simulink model "EKF_SIL_02_newdelIps"  (R2015a)
settings: Solver=ode45  StartTime=0.0  StopTime=totalSimulationTime  RelTol=1e-3
model workspace: external: MATLAB File Init_Model_02_Simulink_SIL1.m (data not in the file)
values from neighbouring files (symbols this model uses):
  Cov_nu = [0.005 0 0 0 ... (first row only)    [InitOOSM.m]    (also in InitSIL.m; Init_Model_02_Simulink.m; Init_Model_02_Simulink_SIL1.m)
  Cov_r = [0.003 0 0 ... (first row only)    [InitOOSM.m]    (also in InitSIL.m; Init_Model_02_Simulink.m; Init_Model_02_Simulink_SIL1.m)
  e_force_x = 0    [InitOOSM.m]    (also in InitSIL.m; Init_Model_02_Simulink.m; Init_Model_02_Simulink_SIL1.m)
  e_force_y = 0    [InitOOSM.m]    (also in InitSIL.m; Init_Model_02_Simulink.m; Init_Model_02_Simulink_SIL1.m)
  e_force_z = 0    [InitOOSM.m]    (also in InitSIL.m; Init_Model_02_Simulink.m; Init_Model_02_Simulink_SIL1.m)
  ieps = [-0.7071;0;0;0.7071]    [InitOOSM.m]    (also in InitSIL.m; Init_Model_02_Simulink.m = [-0.7071; 0; 0; 0.7071]; Init_Model_02_Simulink_SIL1.m)
  ita = [0.5;0.5;0.5;0.5]    [InitOOSM.m]    (also in InitSIL.m; Init_Model_02_Simulink.m = [0.5; 0.5; 0.5; 0.5]; Init_Model_02_Simulink_SIL1.m)
  n = 0.00    (= 0)    [InitOOSM.m]    (also in InitSIL.m; Init_Model_02_Simulink.m; Init_Model_02_Simulink_SIL1.m)
  P_0 = 0.5*eye(18,18)    [InitOOSM.m]    (also in InitSIL.m = 0.05*eye(12,12); Init_Model_02_Simulink.m = 0.005*eye(12,12); Init_Model_02_Simulink_SIL1.m = 0.005*eye(12,12))
  p_x = 0.75    [InitOOSM.m]    (also in InitSIL.m; Init_Model_02_Simulink.m; Init_Model_02_Simulink_SIL1.m)
  p_y = 0.125    [InitOOSM.m]    (also in InitSIL.m; Init_Model_02_Simulink.m; Init_Model_02_Simulink_SIL1.m)
  p_z = -0.8    [InitOOSM.m]    (also in InitSIL.m; Init_Model_02_Simulink.m; Init_Model_02_Simulink_SIL1.m)
  parameter_gravitation = 3.986005E+14    (= 398600500000000)    [InitOOSM.m]    (also in InitSIL.m; Init_Model_02_Simulink.m; Init_Model_02_Simulink_SIL1.m)
  rho = [0.04;0;0.3]    [InitOOSM.m]    (also in InitSIL.m; Init_Model_02_Simulink.m = [0.04; 0; 0.3]; Init_Model_02_Simulink_SIL1.m)
  rho_c = [-0.00017;   -0.9780;   -0.1854]    [InitOOSM.m]    (also in InitSIL.m = [0.00036;   -0.9865;   -0.1854]; Init_Model_02_Simulink.m = [0.00036; -0.9865; -0.1854]; Init_Model_02_Simulink_SIL1.m = [0.00036;   -0.9865;   -0.1854])
  sig_f = 2E-6    (= 2e-06)    [InitOOSM.m]    (also in InitSIL.m; Init_Model_02_Simulink.m; Init_Model_02_Simulink_SIL1.m)
  sig_tau = 2.5E-5    (= 2.5e-05)    [InitOOSM.m]    (also in InitSIL.m; Init_Model_02_Simulink.m; Init_Model_02_Simulink_SIL1.m)
  t_delta = 0.2    [InitOOSM.m]    (also in InitSIL.m; Init_Model_02_Simulink.m; Init_Model_02_Simulink_SIL1.m)
  t_Kalman = 0.01    [InitOOSM.m]    (also in InitSIL.m; Init_Model_02_Simulink.m; Init_Model_02_Simulink_SIL1.m)
  t_RobotSense = 0.05    [InitOOSM.m]    (also in InitSIL.m; Init_Model_02_Simulink.m; Init_Model_02_Simulink_SIL1.m)
  tau_1 = 0    [InitOOSM.m]    (also in InitSIL.m; Init_Model_02_Simulink.m; Init_Model_02_Simulink_SIL1.m)
  tau_2 = 0    [InitOOSM.m]    (also in InitSIL.m; Init_Model_02_Simulink.m; Init_Model_02_Simulink_SIL1.m)
  tau_3 = 0    [InitOOSM.m]    (also in InitSIL.m; Init_Model_02_Simulink.m; Init_Model_02_Simulink_SIL1.m)
  U_n_d = Simulink.Signal    [InitOOSM.m]    (also in InitSIL.m; Init_Model_02_Simulink.m; Init_Model_02_Simulink_SIL1.m)
  X_a_0 = [0; 0; 0; 1; 0; 0; 0; 0; 0; 0; 0; 0; 0;0;0;0;0;0;0;1]    [InitOOSM.m]    (also in InitSIL.m = [0; 0; 0; 1; 0; 0; 0; 0; 0; 0; 0; 0; 0]; Init_Model_02_Simulink.m = [0;0;0;0.707000000000000;0.707000000000000;0.200000000000000; Init_Model_02_Simulink_SIL1.m = [0;0;0.707;0.707;0.2;-0.02;0.0001;0.02;-1.80;0.50;-0.05;0.00)
libraries: simulink x5, dspmtrx3 x2, aerolibtransform2 x2, visionsinks x1
(part 4 of 4)

== system EKF_SIL_02_newdelIps/EKF/Predictor/Dynamic Model (Differential equations)2/Dynamic Model (Differential equations)/Orbital Dynamics /norm  ==
  vector : Inport
  Dot Product : DotProduct  InputSameDT=on  OutDataTypeStr=Inherit: Inherit via internal rule
  Sqrt : Sqrt  SaturateOnIntegerOverflow=on
  "norm " : Outport
  wires:
  Sqrt/1 -> "norm "/1
  vector/1 -> Dot Product/1, Dot Product/2
  Dot Product/1 -> Sqrt/1

== system EKF_SIL_02_newdelIps/EKF/Predictor/Dynamic Model (Differential equations)2/Dynamic Model (Differential equations)/Pose Servicer base//EE/Create Skew Symmetric ==
  vector : Inport
  0 : Constant  Value=0
  Create 3x3 matrix : Subsystem
  Demux : Demux  Outputs=3
  Demux1 : Demux  Outputs=3
  Gain : Gain  Gain=-1
  skew symmetric Matrix : Outport
  wires:
  0/1 -> Create 3x3 matrix/1(a11), Create 3x3 matrix/9(a33), Create 3x3 matrix/5(a22)
  Demux/3 -> Create 3x3 matrix/2(a12)
  Demux1/2 -> Create 3x3 matrix/3(a13)
  Demux1/3 -> Create 3x3 matrix/4(a21)
  Demux/1 -> Create 3x3 matrix/6(a23)
  vector/1 -> Demux1/1, Gain/1
  Create 3x3 matrix/1(Matrix) -> skew symmetric Matrix/1
  Gain/1 -> Demux/1
  Demux/2 -> Create 3x3 matrix/7(a31)
  Demux1/1 -> Create 3x3 matrix/8(a32)

== system EKF_SIL_02_newdelIps/EKF/Predictor/Dynamic Model (Differential equations)2/Dynamic Model (Differential equations)/Rotational Dynamics/Create  J ==
  p : Inport
  0 : Constant  Value=0  SampleTime=-1
  1 : Constant  SampleTime=-1
  Create 3x3 matrix : Subsystem
  Fcn : Fcn  Expr=1-u(2)/1+u(1)
  Fcn1 : Fcn  Expr=1+u(3)/1-u(1)
  "J_k " : Outport
  wires:
  1/1 -> Create 3x3 matrix/1(a11)
  Fcn1/1 -> Create 3x3 matrix/9(a33)
  Create 3x3 matrix/1(Matrix) -> "J_k "/1
  0/1 -> Create 3x3 matrix/2(a12), Create 3x3 matrix/3(a13), Create 3x3 matrix/4(a21), Create 3x3 matrix/6(a23), Create 3x3 matrix/7(a31), Create 3x3 matrix/8(a32)
  p/1 -> Fcn/1, Fcn1/1
  Fcn/1 -> Create 3x3 matrix/5(a22)

== system EKF_SIL_02_newdelIps/EKF/Predictor/Dynamic Model (Differential equations)2/Dynamic Model (Differential equations)/Rotational Dynamics/Create Psi ==
  "omega " : Inport
  p : Inport  Port=2
  Create Psi : Concatenate  NumInputs=3
  Demux : Demux  Outputs=3
  Demux1 : Demux  Outputs=3
  Product{,1..5} (6 alike) : Product
  Scope : Scope
      settings: SaveName=ScopeData20
  Psi : Outport
  wires:
  "omega "/1 -> Demux1/1
  Product3/1 -> Product2/2
  Product5/1 -> Product4/2
  Product1/1 -> Product/2
  Product/1 -> Create Psi/1
  Demux/2 -> Product2/1
  Create Psi/1 -> Psi/1, Scope/1
  Demux/1 -> Product/1
  Product2/1 -> Create Psi/2
  Demux1/2 -> Product5/1, Product1/1
  Demux1/1 -> Product3/1, Product5/2
  Product4/1 -> Create Psi/3
  Demux/3 -> Product4/1
  p/1 -> Demux/1
  Demux1/3 -> Product3/2, Product1/2

== system EKF_SIL_02_newdelIps/Plots and display/Create Measurements [Pose]1/Create Measurements [Position]/Create Rotation Matrix /Create Skew Symmetric/Create 3x3 matrix ==
  a11 : Inport
  a12 : Inport  Port=2
  a13 : Inport  Port=3
  a21 : Inport  Port=4
  a22 : Inport  Port=5
  a23 : Inport  Port=6
  a31 : Inport  Port=7
  a32 : Inport  Port=8
  a33 : Inport  Port=9
  Math Function : Math  Operator=transpose  SaturateOnIntegerOverflow=on
  Reshape (9) to [3x3] column-major : Reshape  OutputDimensionality=Customize  OutputDimensions=[3,3]
  Vector Concatenate : Concatenate  NumInputs=9
  Matrix : Outport
  wires:
  a33/1 -> Vector Concatenate/9
  a22/1 -> Vector Concatenate/5
  Vector Concatenate/1 -> Reshape (9) to [3x3] column-major/1
  a11/1 -> Vector Concatenate/1
  a12/1 -> Vector Concatenate/2
  a13/1 -> Vector Concatenate/3
  a23/1 -> Vector Concatenate/6
  a31/1 -> Vector Concatenate/7
  a32/1 -> Vector Concatenate/8
  a21/1 -> Vector Concatenate/4
  Reshape (9) to [3x3] column-major/1 -> Math Function/1
  Math Function/1 -> Matrix/1

== system EKF_SIL_02_newdelIps/Plots and display/Create Measurements [Pose]2/Create Measurements [Position]/Create Rotation Matrix /Create Skew Symmetric/Create 3x3 matrix ==
  a11 : Inport
  a12 : Inport  Port=2
  a13 : Inport  Port=3
  a21 : Inport  Port=4
  a22 : Inport  Port=5
  a23 : Inport  Port=6
  a31 : Inport  Port=7
  a32 : Inport  Port=8
  a33 : Inport  Port=9
  Math Function : Math  Operator=transpose  SaturateOnIntegerOverflow=on
  Reshape (9) to [3x3] column-major : Reshape  OutputDimensionality=Customize  OutputDimensions=[3,3]
  Vector Concatenate : Concatenate  NumInputs=9
  Matrix : Outport
  wires:
  Math Function/1 -> Matrix/1
  Reshape (9) to [3x3] column-major/1 -> Math Function/1
  a21/1 -> Vector Concatenate/4
  a32/1 -> Vector Concatenate/8
  a31/1 -> Vector Concatenate/7
  a23/1 -> Vector Concatenate/6
  a13/1 -> Vector Concatenate/3
  a12/1 -> Vector Concatenate/2
  a11/1 -> Vector Concatenate/1
  Vector Concatenate/1 -> Reshape (9) to [3x3] column-major/1
  a22/1 -> Vector Concatenate/5
  a33/1 -> Vector Concatenate/9

== system EKF_SIL_02_newdelIps/Plots and display/Create Measurements [Pose]2/Create Measurements [Position]/Create Rotation Matrix 1/Create Skew Symmetric/Create 3x3 matrix ==
  a11 : Inport
  a12 : Inport  Port=2
  a13 : Inport  Port=3
  a21 : Inport  Port=4
  a22 : Inport  Port=5
  a23 : Inport  Port=6
  a31 : Inport  Port=7
  a32 : Inport  Port=8
  a33 : Inport  Port=9
  Math Function : Math  Operator=transpose  SaturateOnIntegerOverflow=on
  Reshape (9) to [3x3] column-major : Reshape  OutputDimensionality=Customize  OutputDimensions=[3,3]
  Vector Concatenate : Concatenate  NumInputs=9
  Matrix : Outport
  wires:
  Math Function/1 -> Matrix/1
  Reshape (9) to [3x3] column-major/1 -> Math Function/1
  a21/1 -> Vector Concatenate/4
  a32/1 -> Vector Concatenate/8
  a31/1 -> Vector Concatenate/7
  a23/1 -> Vector Concatenate/6
  a13/1 -> Vector Concatenate/3
  a12/1 -> Vector Concatenate/2
  a11/1 -> Vector Concatenate/1
  Vector Concatenate/1 -> Reshape (9) to [3x3] column-major/1
  a22/1 -> Vector Concatenate/5
  a33/1 -> Vector Concatenate/9

== system EKF_SIL_02_newdelIps/EKF/Measurement Update/Update with K(k) and predict current state/Create H_k/Create Rotation Matrix /Create Skew Symmetric/Create 3x3 matrix ==
  a11 : Inport
  a12 : Inport  Port=2
  a13 : Inport  Port=3
  a21 : Inport  Port=4
  a22 : Inport  Port=5
  a23 : Inport  Port=6
  a31 : Inport  Port=7
  a32 : Inport  Port=8
  a33 : Inport  Port=9
  Math Function : Math  Operator=transpose  SaturateOnIntegerOverflow=on
  Reshape (9) to [3x3] column-major : Reshape  OutputDimensionality=Customize  OutputDimensions=[3,3]
  Vector Concatenate : Concatenate  NumInputs=9
  Matrix : Outport
  wires:
  a33/1 -> Vector Concatenate/9
  a22/1 -> Vector Concatenate/5
  Vector Concatenate/1 -> Reshape (9) to [3x3] column-major/1
  a11/1 -> Vector Concatenate/1
  a12/1 -> Vector Concatenate/2
  a13/1 -> Vector Concatenate/3
  a23/1 -> Vector Concatenate/6
  a31/1 -> Vector Concatenate/7
  a32/1 -> Vector Concatenate/8
  a21/1 -> Vector Concatenate/4
  Reshape (9) to [3x3] column-major/1 -> Math Function/1
  Math Function/1 -> Matrix/1

== system EKF_SIL_02_newdelIps/EKF/Measurement Update/Update with K(k) and predict current state/Create H_k/Create Rotation Matrix 1/Create Skew Symmetric/Create 3x3 matrix ==
  a11 : Inport
  a12 : Inport  Port=2
  a13 : Inport  Port=3
  a21 : Inport  Port=4
  a22 : Inport  Port=5
  a23 : Inport  Port=6
  a31 : Inport  Port=7
  a32 : Inport  Port=8
  a33 : Inport  Port=9
  Math Function : Math  Operator=transpose  SaturateOnIntegerOverflow=on
  Reshape (9) to [3x3] column-major : Reshape  OutputDimensionality=Customize  OutputDimensions=[3,3]
  Vector Concatenate : Concatenate  NumInputs=9
  Matrix : Outport
  wires:
  Math Function/1 -> Matrix/1
  Reshape (9) to [3x3] column-major/1 -> Math Function/1
  a21/1 -> Vector Concatenate/4
  a32/1 -> Vector Concatenate/8
  a31/1 -> Vector Concatenate/7
  a23/1 -> Vector Concatenate/6
  a13/1 -> Vector Concatenate/3
  a12/1 -> Vector Concatenate/2
  a11/1 -> Vector Concatenate/1
  Vector Concatenate/1 -> Reshape (9) to [3x3] column-major/1
  a22/1 -> Vector Concatenate/5
  a33/1 -> Vector Concatenate/9

== system EKF_SIL_02_newdelIps/EKF/Measurement Update/Update with K(k) and predict current state/Create H_k/Create Rotation Matrix 2/Create Skew Symmetric/Create 3x3 matrix ==
  a11 : Inport
  a12 : Inport  Port=2
  a13 : Inport  Port=3
  a21 : Inport  Port=4
  a22 : Inport  Port=5
  a23 : Inport  Port=6
  a31 : Inport  Port=7
  a32 : Inport  Port=8
  a33 : Inport  Port=9
  Math Function : Math  Operator=transpose  SaturateOnIntegerOverflow=on
  Reshape (9) to [3x3] column-major : Reshape  OutputDimensionality=Customize  OutputDimensions=[3,3]
  Vector Concatenate : Concatenate  NumInputs=9
  Matrix : Outport
  wires:
  a33/1 -> Vector Concatenate/9
  a22/1 -> Vector Concatenate/5
  Vector Concatenate/1 -> Reshape (9) to [3x3] column-major/1
  a11/1 -> Vector Concatenate/1
  a12/1 -> Vector Concatenate/2
  a13/1 -> Vector Concatenate/3
  a23/1 -> Vector Concatenate/6
  a31/1 -> Vector Concatenate/7
  a32/1 -> Vector Concatenate/8
  a21/1 -> Vector Concatenate/4
  Reshape (9) to [3x3] column-major/1 -> Math Function/1
  Math Function/1 -> Matrix/1

== system EKF_SIL_02_newdelIps/EKF/Measurement Update/Update with K(k) and predict current state/Create h/Create Rotation Matrix /Create Skew Symmetric/Create 3x3 matrix ==
  a11 : Inport
  a12 : Inport  Port=2
  a13 : Inport  Port=3
  a21 : Inport  Port=4
  a22 : Inport  Port=5
  a23 : Inport  Port=6
  a31 : Inport  Port=7
  a32 : Inport  Port=8
  a33 : Inport  Port=9
  Math Function : Math  Operator=transpose  SaturateOnIntegerOverflow=on
  Reshape (9) to [3x3] column-major : Reshape  OutputDimensionality=Customize  OutputDimensions=[3,3]
  Vector Concatenate : Concatenate  NumInputs=9
  Matrix : Outport
  wires:
  a33/1 -> Vector Concatenate/9
  a22/1 -> Vector Concatenate/5
  Vector Concatenate/1 -> Reshape (9) to [3x3] column-major/1
  a11/1 -> Vector Concatenate/1
  a12/1 -> Vector Concatenate/2
  a13/1 -> Vector Concatenate/3
  a23/1 -> Vector Concatenate/6
  a31/1 -> Vector Concatenate/7
  a32/1 -> Vector Concatenate/8
  a21/1 -> Vector Concatenate/4
  Reshape (9) to [3x3] column-major/1 -> Math Function/1
  Math Function/1 -> Matrix/1

== system EKF_SIL_02_newdelIps/EKF/Measurement Update/Update with K(k) and predict current state/Create h/Create Rotation Matrix 1/Create Skew Symmetric/Create 3x3 matrix ==
  a11 : Inport
  a12 : Inport  Port=2
  a13 : Inport  Port=3
  a21 : Inport  Port=4
  a22 : Inport  Port=5
  a23 : Inport  Port=6
  a31 : Inport  Port=7
  a32 : Inport  Port=8
  a33 : Inport  Port=9
  Math Function : Math  Operator=transpose  SaturateOnIntegerOverflow=on
  Reshape (9) to [3x3] column-major : Reshape  OutputDimensionality=Customize  OutputDimensions=[3,3]
  Vector Concatenate : Concatenate  NumInputs=9
  Matrix : Outport
  wires:
  a33/1 -> Vector Concatenate/9
  a22/1 -> Vector Concatenate/5
  Vector Concatenate/1 -> Reshape (9) to [3x3] column-major/1
  a11/1 -> Vector Concatenate/1
  a12/1 -> Vector Concatenate/2
  a13/1 -> Vector Concatenate/3
  a23/1 -> Vector Concatenate/6
  a31/1 -> Vector Concatenate/7
  a32/1 -> Vector Concatenate/8
  a21/1 -> Vector Concatenate/4
  Reshape (9) to [3x3] column-major/1 -> Math Function/1
  Math Function/1 -> Matrix/1

== system EKF_SIL_02_newdelIps/EKF/Measurement Update/Update with K(k) and predict current state/Create h/Create Rotation Matrix 2/Create Skew Symmetric/Create 3x3 matrix ==
  a11 : Inport
  a12 : Inport  Port=2
  a13 : Inport  Port=3
  a21 : Inport  Port=4
  a22 : Inport  Port=5
  a23 : Inport  Port=6
  a31 : Inport  Port=7
  a32 : Inport  Port=8
  a33 : Inport  Port=9
  Math Function : Math  Operator=transpose  SaturateOnIntegerOverflow=on
  Reshape (9) to [3x3] column-major : Reshape  OutputDimensionality=Customize  OutputDimensions=[3,3]
  Vector Concatenate : Concatenate  NumInputs=9
  Matrix : Outport
  wires:
  Math Function/1 -> Matrix/1
  Reshape (9) to [3x3] column-major/1 -> Math Function/1
  a21/1 -> Vector Concatenate/4
  a32/1 -> Vector Concatenate/8
  a31/1 -> Vector Concatenate/7
  a23/1 -> Vector Concatenate/6
  a13/1 -> Vector Concatenate/3
  a12/1 -> Vector Concatenate/2
  a11/1 -> Vector Concatenate/1
  Vector Concatenate/1 -> Reshape (9) to [3x3] column-major/1
  a22/1 -> Vector Concatenate/5
  a33/1 -> Vector Concatenate/9

== system EKF_SIL_02_newdelIps/EKF/Predictor/Create State error covariance (P)/State Propagation/Create Rotation Matrix 1/Create Skew Symmetric/Create 3x3 matrix ==
  a11 : Inport
  a12 : Inport  Port=2
  a13 : Inport  Port=3
  a21 : Inport  Port=4
  a22 : Inport  Port=5
  a23 : Inport  Port=6
  a31 : Inport  Port=7
  a32 : Inport  Port=8
  a33 : Inport  Port=9
  Math Function : Math  Operator=transpose  SaturateOnIntegerOverflow=on
  Reshape (9) to [3x3] column-major : Reshape  OutputDimensionality=Customize  OutputDimensions=[3,3]
  Vector Concatenate : Concatenate  NumInputs=9
  Matrix : Outport
  wires:
  a33/1 -> Vector Concatenate/9
  a22/1 -> Vector Concatenate/5
  Vector Concatenate/1 -> Reshape (9) to [3x3] column-major/1
  a11/1 -> Vector Concatenate/1
  a12/1 -> Vector Concatenate/2
  a13/1 -> Vector Concatenate/3
  a23/1 -> Vector Concatenate/6
  a31/1 -> Vector Concatenate/7
  a32/1 -> Vector Concatenate/8
  a21/1 -> Vector Concatenate/4
  Reshape (9) to [3x3] column-major/1 -> Math Function/1
  Math Function/1 -> Matrix/1

== system EKF_SIL_02_newdelIps/EKF/Predictor/Dynamic Model (Differential equations)2/Dynamic Model (Differential equations)/Orbital Dynamics /Create Skew Symmetric/Create 3x3 matrix ==
  a11 : Inport
  a12 : Inport  Port=2
  a13 : Inport  Port=3
  a21 : Inport  Port=4
  a22 : Inport  Port=5
  a23 : Inport  Port=6
  a31 : Inport  Port=7
  a32 : Inport  Port=8
  a33 : Inport  Port=9
  Math Function : Math  Operator=transpose  SaturateOnIntegerOverflow=on
  Reshape (9) to [3x3] column-major : Reshape  OutputDimensionality=Customize  OutputDimensions=[3,3]
  Vector Concatenate : Concatenate  NumInputs=9
  Matrix : Outport
  wires:
  a33/1 -> Vector Concatenate/9
  a22/1 -> Vector Concatenate/5
  Vector Concatenate/1 -> Reshape (9) to [3x3] column-major/1
  a11/1 -> Vector Concatenate/1
  a12/1 -> Vector Concatenate/2
  a13/1 -> Vector Concatenate/3
  a23/1 -> Vector Concatenate/6
  a31/1 -> Vector Concatenate/7
  a32/1 -> Vector Concatenate/8
  a21/1 -> Vector Concatenate/4
  Reshape (9) to [3x3] column-major/1 -> Math Function/1
  Math Function/1 -> Matrix/1

== system EKF_SIL_02_newdelIps/EKF/Predictor/Dynamic Model (Differential equations)2/Dynamic Model (Differential equations)/Pose Servicer base//EE/Create Skew Symmetric/Create 3x3 matrix ==
  a11 : Inport
  a12 : Inport  Port=2
  a13 : Inport  Port=3
  a21 : Inport  Port=4
  a22 : Inport  Port=5
  a23 : Inport  Port=6
  a31 : Inport  Port=7
  a32 : Inport  Port=8
  a33 : Inport  Port=9
  Math Function : Math  Operator=transpose  SaturateOnIntegerOverflow=on
  Reshape (9) to [3x3] column-major : Reshape  OutputDimensionality=Customize  OutputDimensions=[3,3]
  Vector Concatenate : Concatenate  NumInputs=9
  Matrix : Outport
  wires:
  a33/1 -> Vector Concatenate/9
  a22/1 -> Vector Concatenate/5
  Vector Concatenate/1 -> Reshape (9) to [3x3] column-major/1
  a11/1 -> Vector Concatenate/1
  a12/1 -> Vector Concatenate/2
  a13/1 -> Vector Concatenate/3
  a23/1 -> Vector Concatenate/6
  a31/1 -> Vector Concatenate/7
  a32/1 -> Vector Concatenate/8
  a21/1 -> Vector Concatenate/4
  Reshape (9) to [3x3] column-major/1 -> Math Function/1
  Math Function/1 -> Matrix/1

== system EKF_SIL_02_newdelIps/EKF/Predictor/Dynamic Model (Differential equations)2/Dynamic Model (Differential equations)/Rotational Dynamics/Create  J/Create 3x3 matrix ==
  a11 : Inport
  a12 : Inport  Port=2
  a13 : Inport  Port=3
  a21 : Inport  Port=4
  a22 : Inport  Port=5
  a23 : Inport  Port=6
  a31 : Inport  Port=7
  a32 : Inport  Port=8
  a33 : Inport  Port=9
  Math Function : Math  Operator=transpose  SaturateOnIntegerOverflow=on
  Reshape (9) to [3x3] column-major : Reshape  OutputDimensionality=Customize  OutputDimensions=[3,3]
  Vector Concatenate : Concatenate  NumInputs=9
  Matrix : Outport
  wires:
  a33/1 -> Vector Concatenate/9
  a22/1 -> Vector Concatenate/5
  Vector Concatenate/1 -> Reshape (9) to [3x3] column-major/1
  a11/1 -> Vector Concatenate/1
  a12/1 -> Vector Concatenate/2
  a13/1 -> Vector Concatenate/3
  a23/1 -> Vector Concatenate/6
  a31/1 -> Vector Concatenate/7
  a32/1 -> Vector Concatenate/8
  a21/1 -> Vector Concatenate/4
  Reshape (9) to [3x3] column-major/1 -> Math Function/1
  Math Function/1 -> Matrix/1

== matlab function EKF_SIL_02_newdelIps/EKF/Measurement Update/Update with K(k) and predict current state/Create observation/MATLAB Function4 ==
  data: q input; CrossTensor output; flag input
%Inputs: q: quaternion vector
%        flag:0-cross;1-star
function CrossTensor  = fn_CrossTensor(q,flag)
    %#codegen
    CrossTensor = zeros(4,4);
    q_v = q(1:3);
    q_0 = q(4);    
    cross_q_v = fn_VectorToSkewSymmetricTensor(q_v);
    switch (flag)
        case 0
            CrossTensor = [-cross_q_v + q_0*eye(3,3), q_v;-q_v',q_0];
        case 1
            CrossTensor = [cross_q_v + q_0*eye(3,3), q_v;-q_v',q_0];
        otherwise
            
    end
end

== matlab function EKF_SIL_02_newdelIps/Plant/Dynamic Model (Differential equations)/Quaternion Kinematics/MATLAB Function ==
  data: q input; CrossTensor output; flag input
%Inputs: q: quaternion vector
%        flag:0-cross;1-star
function CrossTensor  = fn_CrossTensor(q,flag)
    %#codegen
    CrossTensor = zeros(4,4);
    q_v = q(1:3);
    q_0 = q(4);    
    cross_q_v = fn_VectorToSkewSymmetricTensor(q_v);
    switch (flag)
        case 0
            CrossTensor = [-cross_q_v + q_0*eye(3,3), q_v;-q_v',q_0];
        case 1
            CrossTensor = [cross_q_v + q_0*eye(3,3), q_v;-q_v',q_0];
        otherwise
            
    end
end

== matlab function EKF_SIL_02_newdelIps/Plots and display/Create Measurements [Pose]2/Create Measurements [Orientation] /MATLAB Function1 ==
  data: q input; CrossTensor output; flag input
%Inputs: q: quaternion vector
%        flag:0-cross;1-star
function CrossTensor  = fn_CrossTensor(q,flag)
    %#codegen
    CrossTensor = zeros(4,4);
    q_v = q(1:3);
    q_0 = q(4);    
    cross_q_v = fn_VectorToSkewSymmetricTensor(q_v);
    switch (flag)
        case 0
            CrossTensor = [-cross_q_v + q_0*eye(3,3), q_v;-q_v',q_0];
        case 1
            CrossTensor = [cross_q_v + q_0*eye(3,3), q_v;-q_v',q_0];
        otherwise
            
    end
end

== matlab function EKF_SIL_02_newdelIps/EKF/Create nominal q/MATLAB Function ==
  data: q input; CrossTensor output; flag input
%Inputs: q: quaternion vector
%        flag:0-cross;1-star
function CrossTensor  = fn_CrossTensor(q,flag)
    %#codegen
    CrossTensor = zeros(4,4);
    q_v = q(1:3);
    q_0 = q(4);    
    cross_q_v = fn_VectorToSkewSymmetricTensor(q_v);
    switch (flag)
        case 0
            CrossTensor = [-cross_q_v + q_0*eye(3,3), q_v;-q_v',q_0];
        case 1
            CrossTensor = [cross_q_v + q_0*eye(3,3), q_v;-q_v',q_0];
        otherwise
            
    end
end

== matlab function EKF_SIL_02_newdelIps/EKF/Measurement Update/Create X from X_a/Create del_q [body]/MATLAB Function ==
  data: q input; CrossTensor output; flag input
%Inputs: q: quaternion vector
%        flag:0-cross;1-star
function CrossTensor  = fn_CrossTensor(q,flag)
    %#codegen
    CrossTensor = zeros(4,4);
    q_v = q(1:3);
    q_0 = q(4);    
    cross_q_v = fn_VectorToSkewSymmetricTensor(q_v);
    switch (flag)
        case 0
            CrossTensor = [-cross_q_v + q_0*eye(3,3), q_v;-q_v',q_0];
        case 1
            CrossTensor = [cross_q_v + q_0*eye(3,3), q_v;-q_v',q_0];
        otherwise
            
    end
end

== matlab function EKF_SIL_02_newdelIps/EKF/Predictor/Create State error covariance (P)/State Propagation/MATLAB Function ==
  data: X_a input; Phi output; n input; t_Kalman input; p input; M input; V input; om_EE input
%Function: fn_Create_Phi()
%Inputs: X_a - 23-state vector,
%        n - angular velocity of spacecrafts,
%        t_delta - sampling time
%Outputs: [Phi] (State-propagation Matrix)
%Functionality: Generates the State Propagation matrix
%Author: Hrishik Mishra
function Phi  = fn_Create_Phi(X_a,n,t_Kalman,p,M,V,om_EE)
    Phi_t = fn_Create_Phi_t(n,t_Kalman);
    Phi_r = fn_Create_Phi_r(X_a,p, t_Kalman);    
    Phi_rho_c = expm(fn_VectorToSkewSymmetricTensor(V(4:6))*t_Kalman);
    Phi_ieps = expm(-fn_VectorToSkewSymmetricTensor(om_EE*t_Kalman));
    Phi_robot = [Phi_rho_c,zeros(3,3);zeros(3,3),Phi_ieps];
    
    Phi = [Phi_r, zeros(6,12);zeros(6,6),Phi_t,zeros(6,6);zeros(6,12),Phi_robot];

end
%Create state propagation matrix of the whole system

%Function: fn_Create_Phi_r()
%Inputs: X_a - 23-state vector,
%Outputs: [Phi_r] (State-propagation Matrix for Rotation component)
%Functionality: Generates the State Propagation matrix for Rotation
%component
%Author: Hrishik Mishra
function [Phi_r] = fn_Create_Phi_r(X_a,p,t_Kalman) 
    Phi_r = zeros(6,6);
    omega = X_a(5:7);
    M = fn_Create_M(p,omega);   
    
    A = [-fn_VectorToSkewSymmetricTensor(omega),0.5*eye(3,3);zeros(3,3),M];
    Phi_r = expm(A*t_Kalman);
%     phi_r11 = fn_Create_phi_r11(omega,t_delta);
%     phi_r12 = fn_Create_phi_r12(omega,M,t_delta);
%     phi_r22 = fn_Create_phi_r22(omega,t_delta,M);
%     phi_r13 = fn_Create_phi_r13(omega,t_delta,M,N);
%     phi_r23 = fn_Create_phi_r23(omega,t_delta,M,N);
%     Phi_r = [phi_r11, phi_r12, phi_r13;zeros(3,3),phi_r22,phi_r23;zeros(3,3),zeros(3,3),eye(3,3)];
%     

end
%Function: fn_Create_M()
%Inputs: p - Inertial ratios 
%        omega - angular velocity between Chaser Grasping frame and Chaser
%        CoM
%Outputs: M (Linearized model matrix for inertial parameters)
%Functionality: Generates M
%Author: Hrishik Mishra
function M = fn_Create_M(p,omega)
    %#Codegen
    
    M = [0, p(1)*omega(3), p(1)*omega(2); p(2)*omega(3), 0, p(2)*omega(1); p(3)*omega(2),p(3)*omega(1),0];
end
%Function: fn_Create_N()
%Inputs: omega - angular velocity between Chaser Grasping frame and Chaser
%        CoM
%Outputs: N (Linearized model matrix for inertial parameters)
%Functionality: Generates M
%Author: Hrishik Mishra
function N = fn_Create_N(omega)
%
    N = [omega(2)*omega(3), 0, 0; 0, omega(1)*omega(3), 0; 0, 0, omega(1)*omega(2)];
end

%%
%Function: fn_Create_Phi_t()
%Inputs: n - angular velocity of Chaser/Target (almost same)
%        t_delta - sampling time
%Outputs: Phi_t (State Transition Matrix for Translation component)
%Functionality: Generates Phi_t
%Author: Hrishik Mishra
function Phi_t = fn_Create_Phi_t(n,t_delta)
%
    Phi_t12 = [t_delta, n*t_delta^2,0;0, t_delta, 0;0,0,t_delta];
    Phi_t22 = eye(3,3) - 2*fn_VectorToSkewSymmetricTensor([0;0;n])*t_delta;
    
    Phi_t = [eye(3,3),Phi_t12;zeros(3,3),Phi_t22];
    
end

== matlab function EKF_SIL_02_newdelIps/EKF/Predictor/Create State error covariance (P)/Process noise covariance [rotational]/Process Noise covariance ==
  data: Phi input; Q_r output; unused1 input; t_delta input; tau input; unused input; p input
%Function: fn_Create_Q_r()
%Inputs: Phi - State Propagation Matrix for Rotational component
%        X - 23-state vector
%        t_delta - sampling time
%        tau - Torque disturbance
%        sig_p - Uncertainty in Inertial ratios (p)
%Outputs: Q_r (Rotation component Process noise)
%Functionality: Generates Q_r
%Author: Hrishik Mishra
function Q_r = fn_Create_Q_r(Phi,~, t_delta, tau,~,p)
    %#codegen
    J = fn_Create_J(p);
    Q_r11 = 0.25*fn_Create_Q_r11(Phi(1:3,4:6), J, t_delta, tau);
    Q_r12 = 0.5*fn_Create_Q_r12(Phi(1:3,4:6),Phi(4:6,4:6),J,t_delta,tau);
    Q_r22 = fn_Create_Q_r22(Phi(4:6,4:6),J,t_delta,tau);
    Q_r = [Q_r11, Q_r12;Q_r12' Q_r22];
    
end
%check if it is actually phi_r12 or phi_r11
function Q_r11 = fn_Create_Q_r11(phi_r12, J, t_delta, tau)
    Q_r11 = tau*phi_r12*J^2*phi_r12'*t_delta; 
end

function Q_r12 = fn_Create_Q_r12(phi_r12,phi_r22,J, t_delta, tau)
    Q_r12 = tau*phi_r12*J^2*phi_r22*t_delta;
end
function Q_r22 = fn_Create_Q_r22(phi_r22, J, t_delta, tau)
    Q_r22 = tau*phi_r22*J^2*phi_r22*t_delta;
end
%Function: fn_Create_J()
%Inputs: p: Inertial ratios
%Outputs: J (Inertial Ratio Matrix for omega_dot)
%Functionality: Generates J
%Author: Hrishik Mishra
function J = fn_Create_J(p)
    J = [1 0 0;0 (1-p(2))/(1+p(1)) 0;0 0 (1+p(3))/(1-p(1))];
end

== matlab function EKF_SIL_02_newdelIps/EKF/Predictor/Create State error covariance (P)/Process noise covariance [translational]/Process noise covariance [translational] ==
  data: t_Kalman input; Q_t_k output; n input; sigma_f input
%Function: fn_Create_Q_t_k()
%Inputs: t_delta: sampling time
%        sigma_f: variance of force perturbations
%Outputs: Q_t_k (Translational component Process noise)
%Functionality: Generates Q_t_k
%Author: Hrishik Mishra
function Q_t_k  = fn_Create_Q_t_k(t_Kalman, n,sigma_f)
    %#codegen

    Q_t11_k = [(t_Kalman^3)/3 + (2/5)*n^2*t_Kalman^5, (1/4)*(n - n^2)*t_Kalman^4, 0;(1/4)*(n - n^2)*t_Kalman^4, (t_Kalman^3)/3 - (4/15)*n^2*t_Kalman^5 0;0, 0, (t_Kalman^3)/3 - (1/15)*n^2*t_Kalman^5];
    Q_t12_k = [(t_Kalman^2)/2 + (1/3)*(n^2)*(t_Kalman^4), -(1/3)*n*(t_Kalman^3),0;(2/3)*(n - n^2)*t_Kalman^3, (1/2)*(t_Kalman^2) - (2/3)*(n^2)*(t_Kalman^4) 0;0 0 (1/2)*(t_Kalman^2) - (1/6)*(n^2)*(t_Kalman^4)];
    Q_t22_k = [t_Kalman + (n^2)*(t_Kalman^3), 0, 0;0, t_Kalman, 0;0, 0, t_Kalman - (1/3)*(n^2)*(t_Kalman^3)];

    Q_t_k = [Q_t11_k, Q_t12_k;Q_t12_k',Q_t22_k];

    Q_t_k = sigma_f*Q_t_k;
end

== matlab function EKF_SIL_02_newdelIps/EKF/Measurement Update/Update with K(k) and predict current state/Create H_k/MATLAB Function2 ==
  data: q input; CrossTensor output; flag input
%Inputs: q: quaternion vector
%        flag:0-cross;1-star
function CrossTensor  = fn_CrossTensor(q,flag)
    %#codegen
    CrossTensor = zeros(4,4);
    q_v = q(1:3);
    q_0 = q(4);    
    cross_q_v = fn_VectorToSkewSymmetricTensor(q_v);
    switch (flag)
        case 0
            CrossTensor = [-cross_q_v + q_0*eye(3,3), q_v;-q_v',q_0];
        case 1
            CrossTensor = [cross_q_v + q_0*eye(3,3), q_v;-q_v',q_0];
        otherwise
            
    end
end

== matlab function EKF_SIL_02_newdelIps/EKF/Measurement Update/Update with K(k) and predict current state/Create S_k/Measurement noise covariance ==
  data: q_nominal input; S output; ita_nominal input; cov_r input; cov_nu input; trig_1 input; trig_2 input
%Function: fn_Create_S()
%Inputs: q_nominal: Quaternion between Chaser CoM and Target CoM
%        ita_nominal: Quaternion between Target CoM and Target grasping
%        frame
%        cov_r: position covariance due to camera
%        cov_nu: orientation covariance due to camera
%Outputs: S (Measurement noise covariance Matrix)
%Functionality: Generates S
%Author: Hrishik Mishra
function S  = fn_Create_S(q_nominal,ita_nominal,cov_r,cov_nu,trig_1,trig_2)
    %#codegen
    q_star = [-q_nominal(1:3);q_nominal(4)];
    ita_star = [-ita_nominal(1:3);ita_nominal(4)];
    Ita_Tensor = fn_CrossTensor(ita_star,0);
    Q_Tensor = fn_CrossTensor(q_star,1);
    T = [eye(3,3),zeros(3,1)]*Ita_Tensor*Q_Tensor;
    S_cam = [cov_r,zeros(3,3);zeros(3,3), T*cov_nu*T'];
    S = S_cam;
    %S = 1e-14*eye(6,6);
end

== matlab function EKF_SIL_02_newdelIps/EKF/Measurement Update/Update with K(k) and predict current state/Create observation/MATLAB Function2 ==
  data: q input; CrossTensor output; flag input
%Inputs: q: quaternion vector
%        flag:0-cross;1-star
function CrossTensor  = fn_CrossTensor(q,flag)
    %#codegen
    CrossTensor = zeros(4,4);
    q_v = q(1:3);
    q_0 = q(4);    
    cross_q_v = fn_VectorToSkewSymmetricTensor(q_v);
    switch (flag)
        case 0
            CrossTensor = [-cross_q_v + q_0*eye(3,3), q_v;-q_v',q_0];
        case 1
            CrossTensor = [cross_q_v + q_0*eye(3,3), q_v;-q_v',q_0];
        otherwise
            
    end
end

== matlab function EKF_SIL_02_newdelIps/EKF/Measurement Update/Update with K(k) and predict current state/Create h/MATLAB Function2 ==
  data: q input; CrossTensor output; flag input
%Inputs: q: quaternion vector
%        flag:0-cross;1-star
function CrossTensor  = fn_CrossTensor(q,flag)
    %#codegen
    CrossTensor = zeros(4,4);
    q_v = q(1:3);
    q_0 = q(4);    
    cross_q_v = fn_VectorToSkewSymmetricTensor(q_v);
    switch (flag)
        case 0
            CrossTensor = [-cross_q_v + q_0*eye(3,3), q_v;-q_v',q_0];
        case 1
            CrossTensor = [cross_q_v + q_0*eye(3,3), q_v;-q_v',q_0];
        otherwise
            
    end
end

== matlab function EKF_SIL_02_newdelIps/EKF/Measurement Update/Update with K(k) and predict current state/Create X_a from X/Create q_nominal /MATLAB Function2 ==
  data: q input; CrossTensor output; flag input
%Inputs: q: quaternion vector
%        flag:0-cross;1-star
function CrossTensor  = fn_CrossTensor(q,flag)
    %#codegen
    CrossTensor = zeros(4,4);
    q_v = q(1:3);
    q_0 = q(4);    
    cross_q_v = fn_VectorToSkewSymmetricTensor(q_v);
    switch (flag)
        case 0
            CrossTensor = [-cross_q_v + q_0*eye(3,3), q_v;-q_v',q_0];
        case 1
            CrossTensor = [cross_q_v + q_0*eye(3,3), q_v;-q_v',q_0];
        otherwise
            
    end
end

== matlab function EKF_SIL_02_newdelIps/EKF/Measurement Update/Update with K(k) and predict current state/Create observation/MATLAB Function5 ==
  data: q input; CrossTensor output; flag input
%Inputs: q: quaternion vector
%        flag:0-cross;1-star
function CrossTensor  = fn_CrossTensor(q,flag)
    %#codegen
    CrossTensor = zeros(4,4);
    q_v = q(1:3);
    q_0 = q(4);    
    cross_q_v = fn_VectorToSkewSymmetricTensor(q_v);
    switch (flag)
        case 0
            CrossTensor = [-cross_q_v + q_0*eye(3,3), q_v;-q_v',q_0];
        case 1
            CrossTensor = [cross_q_v + q_0*eye(3,3), q_v;-q_v',q_0];
        otherwise
            
    end
end

== matlab function EKF_SIL_02_newdelIps/Plots and display/Create Measurements [Pose]1/Create Measurements [Orientation] /MATLAB Function ==
  data: q input; CrossTensor output; flag input
%Inputs: q: quaternion vector
%        flag:0-cross;1-star
function CrossTensor  = fn_CrossTensor(q,flag)
    %#codegen
    CrossTensor = zeros(4,4);
    q_v = q(1:3);
    q_0 = q(4);    
    cross_q_v = fn_VectorToSkewSymmetricTensor(q_v);
    switch (flag)
        case 0
            CrossTensor = [-cross_q_v + q_0*eye(3,3), q_v;-q_v',q_0];
        case 1
            CrossTensor = [cross_q_v + q_0*eye(3,3), q_v;-q_v',q_0];
        otherwise
            
    end
end

== matlab function EKF_SIL_02_newdelIps/EKF/Measurement Update/Update with K(k) and predict current state/Create h/Subsystem2/MATLAB Function2 ==
  data: q input; CrossTensor output; flag input
%Inputs: q: quaternion vector
%        flag:0-cross;1-star
function CrossTensor  = fn_CrossTensor(q,flag)
    %#codegen
    CrossTensor = zeros(4,4);
    q_v = q(1:3);
    q_0 = q(4);    
    cross_q_v = fn_VectorToSkewSymmetricTensor(q_v);
    switch (flag)
        case 0
            CrossTensor = [-cross_q_v + q_0*eye(3,3), q_v;-q_v',q_0];
        case 1
            CrossTensor = [cross_q_v + q_0*eye(3,3), q_v;-q_v',q_0];
        otherwise
            
    end
end

== matlab function EKF_SIL_02_newdelIps/EKF/Measurement Update/Update with K(k) and predict current state/Kalman gain/MATLAB Function ==
  data: H input size=[12,18]; K output size=[18,12]; P_pre input; S_k input size=[12,12]; Cov_x_y output size=[12,12]
function [K,Cov_x_y] = fcn(H,P_pre,S_k)
%#codegen
    coder.varsize('K_temp',[18,12],[0,1]);
    coder.varsize('Cov_x_y',[12,12],[1,1]);
    %coder.varsize('H',[12,18],[1,0]);
    coder.varsize('Sk',[12,12],[1,1]);
    K_temp = P_pre*H'*inv(H*P_pre*H' + S_k);
    K = K_temp(1:18,:);
    Cov_x_y = H*P_pre*H' + S_k;
end

== matlab function EKF_SIL_02_newdelIps/EKF/Predictor/Dynamic Model (Differential equations)2/Dynamic Model (Differential equations)/Quaternion Kinematics/MATLAB Function ==
  data: q input; CrossTensor output; flag input
%Inputs: q: quaternion vector
%        flag:0-cross;1-star
function CrossTensor  = fn_CrossTensor(q,flag)
    %#codegen
    CrossTensor = zeros(4,4);
    q_v = q(1:3);
    q_0 = q(4);    
    cross_q_v = fn_VectorToSkewSymmetricTensor(q_v);
    switch (flag)
        case 0
            CrossTensor = [-cross_q_v + q_0*eye(3,3), q_v;-q_v',q_0];
        case 1
            CrossTensor = [cross_q_v + q_0*eye(3,3), q_v;-q_v',q_0];
        otherwise
            
    end
end

== matlab function EKF_SIL_02_newdelIps/Plots and display/Create Measurements [Pose]2/Create Measurements [Orientation] /MATLAB Function ==
  data: q input; CrossTensor output; flag input
%Inputs: q: quaternion vector
%        flag:0-cross;1-star
function CrossTensor  = fn_CrossTensor(q,flag)
    %#codegen
    CrossTensor = zeros(4,4);
    q_v = q(1:3);
    q_0 = q(4);    
    cross_q_v = fn_VectorToSkewSymmetricTensor(q_v);
    switch (flag)
        case 0
            CrossTensor = [-cross_q_v + q_0*eye(3,3), q_v;-q_v',q_0];
        case 1
            CrossTensor = [cross_q_v + q_0*eye(3,3), q_v;-q_v',q_0];
        otherwise
            
    end
end

== matlab function EKF_SIL_02_newdelIps/EKF/Measurement Update/Update with K(k) and predict current state/Create observation/MATLAB Function1 ==
  data: q input; CrossTensor output; flag input
%Inputs: q: quaternion vector
%        flag:0-cross;1-star
function CrossTensor  = fn_CrossTensor(q,flag)
    %#codegen
    CrossTensor = zeros(4,4);
    q_v = q(1:3);
    q_0 = q(4);    
    cross_q_v = fn_VectorToSkewSymmetricTensor(q_v);
    switch (flag)
        case 0
            CrossTensor = [-cross_q_v + q_0*eye(3,3), q_v;-q_v',q_0];
        case 1
            CrossTensor = [cross_q_v + q_0*eye(3,3), q_v;-q_v',q_0];
        otherwise
            
    end
end

== matlab function EKF_SIL_02_newdelIps/EKF/Measurement Update/Update with K(k) and predict current state/K*H/MATLAB Function ==
  data: K input; y output size=[18,18]; H input
function y = fcn(K,H)
%#codegen
    assert(size(K*H,1)==18 && size(K*H,1)==18);
    coder.varsize('y',[18,18],[0,0]);
    temp = K*H;
    y = temp(1:18,1:18);
end

== matlab function EKF_SIL_02_newdelIps/EKF/Measurement Update/Update with K(k) and predict current state/Subsystem/MATLAB Function ==
  data: K input size=[18,12]; y output; del_x input size=[12]
function y = fcn(K,del_x)
%#codegen      
    coder.varsize('temp',18,1);
    temp = K*del_x;
    assert(size(temp,1)==18 && size(temp,2)==1);
    y = temp(1:18,1);
end

== matlab function EKF_SIL_02_newdelIps/EKF/Measurement Update/Update with K(k) and predict current state/MhDist/MATLAB Function ==
  data: x input size=12; y output; Var input size=[12,12]
function y = fcn(x,Var)
%#codegen
    y = x'*inv(Var)*x;
end

== matlab function EKF_SIL_02_newdelIps/EKF/Measurement Update/Update with K(k) and predict current state/Create H_k/MATLAB Function ==
  data: u input size=[12,18]; y output size=[12,18]
function y = fcn(u)
%#codegen
coder.varsize('y_temp',[12,18],[1,0]);
y_temp = u;
assert(size(y_temp,2) == 18);
y = y_temp(:,1:18);

== matlab function EKF_SIL_02_newdelIps/EKF/Measurement Update/Update with K(k) and predict current state/Create h/Subsystem1/MATLAB Function2 ==
  data: q input; CrossTensor output; flag input
%Inputs: q: quaternion vector
%        flag:0-cross;1-star
function CrossTensor  = fn_CrossTensor(q,flag)
    %#codegen
    CrossTensor = zeros(4,4);
    q_v = q(1:3);
    q_0 = q(4);    
    cross_q_v = fn_VectorToSkewSymmetricTensor(q_v);
    switch (flag)
        case 0
            CrossTensor = [-cross_q_v + q_0*eye(3,3), q_v;-q_v',q_0];
        case 1
            CrossTensor = [cross_q_v + q_0*eye(3,3), q_v;-q_v',q_0];
        otherwise
            
    end
end

== matlab function EKF_SIL_02_newdelIps/EKF/Measurement Update/Update with K(k) and predict current state/Create observation/MATLAB Function3 ==
  data: q input; CrossTensor output; flag input
%Inputs: q: quaternion vector
%        flag:0-cross;1-star
function CrossTensor  = fn_CrossTensor(q,flag)
    %#codegen
    CrossTensor = zeros(4,4);
    q_v = q(1:3);
    q_0 = q(4);    
    cross_q_v = fn_VectorToSkewSymmetricTensor(q_v);
    switch (flag)
        case 0
            CrossTensor = [-cross_q_v + q_0*eye(3,3), q_v;-q_v',q_0];
        case 1
            CrossTensor = [cross_q_v + q_0*eye(3,3), q_v;-q_v',q_0];
        otherwise
            
    end
end

== matlab function EKF_SIL_02_newdelIps/EKF/Measurement Update/Update with K(k) and predict current state/Create X_a from X/Create ieps /MATLAB Function2 ==
  data: q input; CrossTensor output; flag input
%Inputs: q: quaternion vector
%        flag:0-cross;1-star
function CrossTensor  = fn_CrossTensor(q,flag)
    %#codegen
    CrossTensor = zeros(4,4);
    q_v = q(1:3);
    q_0 = q(4);    
    cross_q_v = fn_VectorToSkewSymmetricTensor(q_v);
    switch (flag)
        case 0
            CrossTensor = [-cross_q_v + q_0*eye(3,3), q_v;-q_v',q_0];
        case 1
            CrossTensor = [cross_q_v + q_0*eye(3,3), q_v;-q_v',q_0];
        otherwise
            
    end
end

== matlab function EKF_SIL_02_newdelIps/EKF/Predictor/Dynamic Model (Differential equations)2/Dynamic Model (Differential equations)/Pose Servicer base//EE/MATLAB Function1 ==
  data: q input; CrossTensor output; flag input
%Inputs: q: quaternion vector
%        flag:0-cross;1-star
function CrossTensor  = fn_CrossTensor(q,flag)
    %#codegen
    CrossTensor = zeros(4,4);
    q_v = q(1:3);
    q_0 = q(4);    
    cross_q_v = fn_VectorToSkewSymmetricTensor(q_v);
    switch (flag)
        case 0
            CrossTensor = [-cross_q_v + q_0*eye(3,3), q_v;-q_v',q_0];
        case 1
            CrossTensor = [cross_q_v + q_0*eye(3,3), q_v;-q_v',q_0];
        otherwise
            
    end
end

== matlab function EKF_SIL_02_newdelIps/EKF/Measurement Update/Create X from X_a/Create del_q [inertial]/MATLAB Function ==
  data: q input; CrossTensor output; flag input
%Inputs: q: quaternion vector
%        flag:0-cross;1-star
function CrossTensor  = fn_CrossTensor(q,flag)
    %#codegen
    CrossTensor = zeros(4,4);
    q_v = q(1:3);
    q_0 = q(4);    
    cross_q_v = fn_VectorToSkewSymmetricTensor(q_v);
    switch (flag)
        case 0
            CrossTensor = [-cross_q_v + q_0*eye(3,3), q_v;-q_v',q_0];
        case 1
            CrossTensor = [cross_q_v + q_0*eye(3,3), q_v;-q_v',q_0];
        otherwise
            
    end
end

== matlab function EKF_SIL_02_newdelIps/EKF/Create nominal q1/MATLAB Function ==
  data: q input; CrossTensor output; flag input
%Inputs: q: quaternion vector
%        flag:0-cross;1-star
function CrossTensor  = fn_CrossTensor(q,flag)
    %#codegen
    CrossTensor = zeros(4,4);
    q_v = q(1:3);
    q_0 = q(4);    
    cross_q_v = fn_VectorToSkewSymmetricTensor(q_v);
    switch (flag)
        case 0
            CrossTensor = [-cross_q_v + q_0*eye(3,3), q_v;-q_v',q_0];
        case 1
            CrossTensor = [cross_q_v + q_0*eye(3,3), q_v;-q_v',q_0];
        otherwise
            
    end
end
